simulink library "performance_model_library"  (R2018b)
settings: Solver=VariableStepAuto  StartTime=0.0  StopTime=10.0  RelTol=1e-3
undefined symbols (not defined in the file): VIS_CAM, VIS_CAM_sensor_time
libraries: vrlib x1
settings Model: Creator=Gaia Civardi  LastModifiedBy=andrea

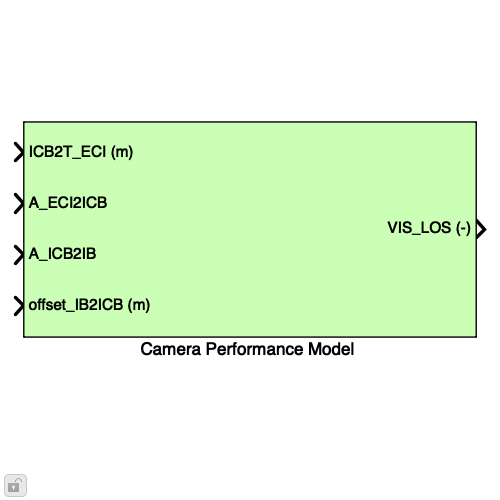
[thumbnail: Simulink's stored preview of the top-level diagram]
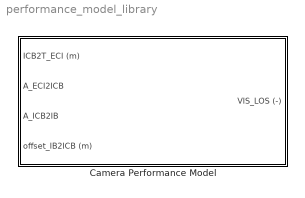
== system performance_model_library ==
  "Camera Performance Model " : Subsystem  mask{CAM=VIS_CAM, sensor_time=VIS_CAM_sensor_time}
      mask prompts: CAM "CAM Data Structure"; sensor_time "Sensor Time (s)"
      mask DialogControl Container4 Prompt: Block Description
      mask DialogControl Control1 Prompt: This block simulates a camera sensors that takes a chaser to target vector in ECI axes and outputs the camera to target Line-of-Sight (LOS) vector, expressed in camera axes. The transformation accounts for the real sensor errors.
      mask DialogControl DescGroupVar Prompt: Parameters

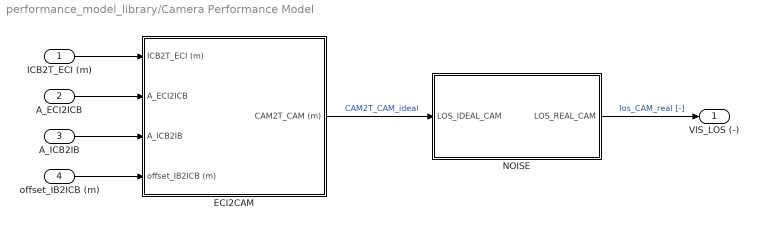
== system performance_model_library/Camera Performance Model  ==
  ICB2T_ECI (m) : Inport
  A_ECI2ICB : Inport  Port=2
  A_ICB2IB : Inport  Port=3
  offset_IB2ICB (m) : Inport  Port=4
  ECI2CAM : Subsystem  mask{DCM_mounterr=CAM.DCM_mounterr, offset_mounterr=CAM.offset_mounterr, A_IB2CAM=CAM.A_IB2CAM, offset_CAM2IB=CAM.offset_CAM2IB}
      mask prompts: DCM_mounterr "Camera DCM Mounting Error"; offset_mounterr "Camera Offset Mounting Error [m]"; A_IB2CAM "Rotation Matrix from IB to CAM"; offset_CAM2IB "Offset (IB-CAM) [m]"
      mask DialogControl Container4 Prompt: Block Description
      mask DialogControl Control1 Prompt: This block convers the chaser to target vector in ECI axes, to a camera to target vector, expressed in the camera axes. The transformation accounts for possible camera mounting errors.
      mask DialogControl DescGroupVar Prompt: Parameters
      mask DialogControl Container2 Prompt: Stochastic Parameters
      mask DialogControl Container3 Prompt: Deterministic Parameters
  NOISE : Subsystem
  " VIS_LOS (-)" : Outport  VectorParamsAs1DForOutWhenUnconnected=off
  wires:
  offset_IB2ICB (m)/1 -> ECI2CAM/4(offset_IB2ICB (m))
  A_ICB2IB/1 -> ECI2CAM/3(A_ICB2IB)
  A_ECI2ICB/1 -> ECI2CAM/2(A_ECI2ICB)
  ICB2T_ECI (m)/1 -> ECI2CAM/1("ICB2T_ECI (m) ")
  NOISE/1("LOS_REAL_CAM ") -> " VIS_LOS (-)"/1  "los_CAM_real [-]"
  ECI2CAM/1(CAM2T_CAM (m)) -> NOISE/1(LOS_IDEAL_CAM)  "CAM2T_CAM_ideal"

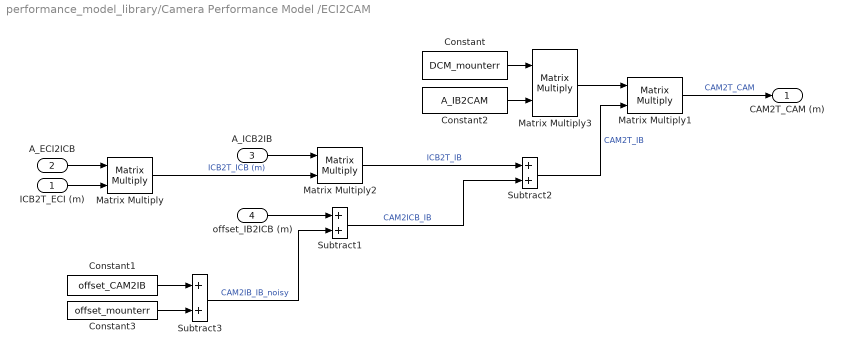
== system performance_model_library/Camera Performance Model /ECI2CAM ==
  "ICB2T_ECI (m) " : Inport
  A_ECI2ICB : Inport  Port=2
  A_ICB2IB : Inport  Port=3
  offset_IB2ICB (m) : Inport  Port=4
  Constant : Constant  Value=DCM_mounterr
  Constant1 : Constant  Value=offset_CAM2IB
  Constant2 : Constant  Value=A_IB2CAM
  Constant3 : Constant  Value=offset_mounterr
  Matrix Multiply{,1..3} (4 alike) : Product  Multiplication=Matrix(*)
  Subtract1 : Sum
  Subtract2 : Sum
  Subtract3 : Sum
  CAM2T_CAM (m) : Outport  VectorParamsAs1DForOutWhenUnconnected=off
  wires:
  Constant3/1 -> Subtract3/2
  Matrix Multiply3/1 -> Matrix Multiply1/1
  Constant/1 -> Matrix Multiply3/1
  Subtract3/1 -> Subtract1/2  "CAM2IB_IB_noisy"
  Constant1/1 -> Subtract3/1
  Subtract1/1 -> Subtract2/2  "CAM2ICB_IB"
  offset_IB2ICB (m)/1 -> Subtract1/1
  Matrix Multiply/1 -> Matrix Multiply2/2  "ICB2T_ICB (m)"
  Matrix Multiply1/1 -> CAM2T_CAM (m)/1  "CAM2T_CAM"
  Matrix Multiply2/1 -> Subtract2/1  "ICB2T_IB"
  A_ICB2IB/1 -> Matrix Multiply2/1
  Subtract2/1 -> Matrix Multiply1/2  "CAM2T_IB"
  "ICB2T_ECI (m) "/1 -> Matrix Multiply/2
  A_ECI2ICB/1 -> Matrix Multiply/1
  Constant2/1 -> Matrix Multiply3/2

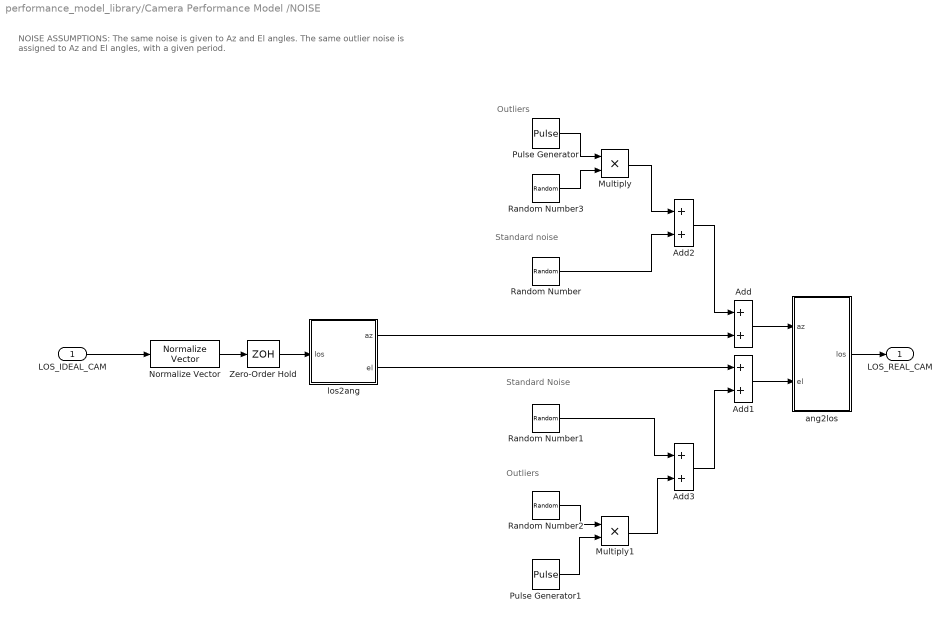
== system performance_model_library/Camera Performance Model /NOISE ==
  note: NOISE ASSUMPTIONS:
      | The same noise is given to Az and El angles.
      | The same outlier noise is assigned to Az and El angles, with a given period.
  note: Standard Noise
  note: Outliers
  note: Standard noise
  note: Outliers
  LOS_IDEAL_CAM : Inport
  Add{,1..3} (4 alike) : Sum
  Multiply : Product
  Multiply1 : Product
  Normalize Vector : vrlib/Utilities/Normalize Vector  maxzero=0
  Pulse Generator : DiscretePulseGenerator  Period=CAM.outlier_period  PulseWidth=CAM.outlier_width  PhaseDelay=CAM.outlier_delay  SampleTime=sensor_time
  Pulse Generator1 : DiscretePulseGenerator  Period=CAM.outlier_period  PulseWidth=CAM.outlier_width  PhaseDelay=CAM.outlier_delay  SampleTime=sensor_time
  Random Number : RandomNumber  Variance=CAM.std_noise^2  Seed=CAM.seed+2  SampleTime=sensor_time
  Random Number1 : RandomNumber  Variance=CAM.std_noise^2  Seed=CAM.seed+3  SampleTime=sensor_time
  Random Number2 : RandomNumber  Variance=CAM.std_outlier_noise^2  Seed=CAM.seed+4  SampleTime=sensor_time
  Random Number3 : RandomNumber  Variance=CAM.std_outlier_noise^2  Seed=CAM.seed+1  SampleTime=sensor_time
  Zero-Order Hold : ZeroOrderHold  SampleTime=sensor_time
  ang2los : Subsystem
  los2ang : Subsystem
  "LOS_REAL_CAM " : Outport  VectorParamsAs1DForOutWhenUnconnected=off
  wires:
  Normalize Vector/1 -> Zero-Order Hold/1
  LOS_IDEAL_CAM/1 -> Normalize Vector/1
  Add/1 -> ang2los/1(az)
  Add1/1 -> ang2los/2(el)
  Zero-Order Hold/1 -> los2ang/1(los)
  ang2los/1(los) -> "LOS_REAL_CAM "/1
  los2ang/1(az) -> Add/2
  los2ang/2(el) -> Add1/1
  Pulse Generator/1 -> Multiply/1
  Random Number3/1 -> Multiply/2
  Multiply/1 -> Add2/1
  Random Number/1 -> Add2/2
  Add2/1 -> Add/1
  Random Number2/1 -> Multiply1/1
  Pulse Generator1/1 -> Multiply1/2
  Random Number1/1 -> Add3/1
  Multiply1/1 -> Add3/2
  Add3/1 -> Add1/2

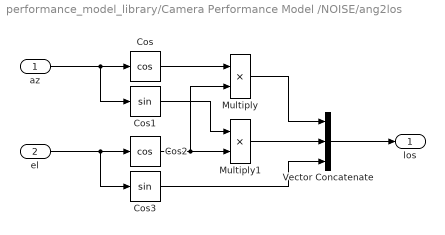
== system performance_model_library/Camera Performance Model /NOISE/ang2los ==
  az : Inport
  el : Inport  Port=2
  Cos : Trigonometry  Operator=cos
  Cos1 : Trigonometry
  Cos2 : Trigonometry  Operator=cos
  Cos3 : Trigonometry
  Multiply : Product
  Multiply1 : Product
  Vector Concatenate : Concatenate  NumInputs=3
  los : Outport  VectorParamsAs1DForOutWhenUnconnected=off
  wires:
  Multiply/1 -> Vector Concatenate/1
  Multiply1/1 -> Vector Concatenate/2
  Cos/1 -> Multiply/1
  Cos3/1 -> Vector Concatenate/3
  Cos2/1 -> Multiply1/2, Multiply/2
  Vector Concatenate/1 -> los/1
  az/1 -> Cos1/1, Cos/1
  Cos1/1 -> Multiply1/1
  el/1 -> Cos2/1, Cos3/1

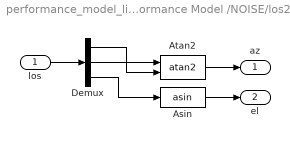
== system performance_model_library/Camera Performance Model /NOISE/los2ang ==
  los : Inport
  Asin : Trigonometry  Operator=asin
  Atan2 : Trigonometry  Operator=atan2
  Demux : Demux  Outputs=3
  az : Outport  VectorParamsAs1DForOutWhenUnconnected=off
  el : Outport  Port=2  VectorParamsAs1DForOutWhenUnconnected=off
  wires:
  los/1 -> Demux/1
  Demux/1 -> Atan2/2
  Demux/3 -> Asin/1
  Atan2/1 -> az/1
  Asin/1 -> el/1
  Demux/2 -> Atan2/1
